simulink model "SolverSS_TestBed"  (R2012b)
settings: Solver=FixedStepDiscrete  StartTime=0.0  StopTime=100  FixedStep=1  RelTol=1e-3
libraries: Lib_Solve_SSNRSolverJC_TMATS x1
settings Model: Creator=jwchapm2  LastModifiedBy=jwchapm2

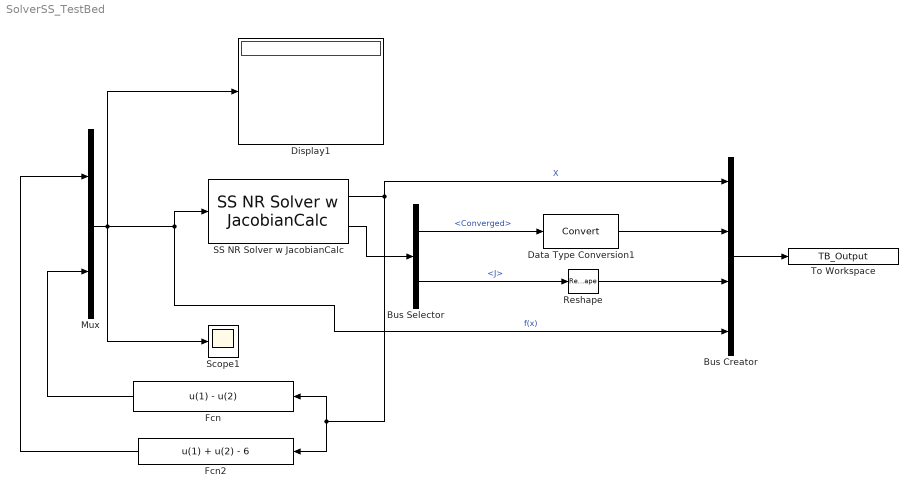
== system SolverSS_TestBed ==
  Bus Creator : BusCreator
  Bus Selector : BusSelector  OutputSignals=Converged,J
  Data Type Conversion1 : DataTypeConversion
  Display1 : Display
  Fcn : Fcn  Expr=u(1) - u(2)
  Fcn2 : Fcn  Expr=u(1) + u(2) - 6
  Mux : Mux  Inputs=2
  Reshape : Reshape
  SS NR Solver w JacobianCalc : Lib_Solve_SSNRSolverJC_TMATS/SS NR Solver w JacobianCalc  SJac_Per_M=MWS.SolverSS.Per  SNR_IC_M=MWS.SolverSS.IC  SNR_DX_M=MWS.SolverSS.dX  SJacobianAttempts_M=MWS.SolverSS.Jatm  Cond_Limits_M=MWS.SolverSS.Cond_Lim
  Scope1 : Scope
  To Workspace : ToWorkspace  VariableName=TB_Output  SampleTime=-1
  wires:
  Mux/1 -> Scope1/1, Display1/1, Bus Creator/4, SS NR Solver w JacobianCalc/1  "f(x)"
  SS NR Solver w JacobianCalc/1 -> Fcn2/1, Fcn/1, Bus Creator/1  "X"
  Bus Creator/1 -> To Workspace/1
  Fcn/1 -> Mux/2
  Fcn2/1 -> Mux/1
  SS NR Solver w JacobianCalc/2 -> Bus Selector/1
  Bus Selector/1 -> Data Type Conversion1/1  "<Converged>"
  Bus Selector/2 -> Reshape/1  "<J>"
  Data Type Conversion1/1 -> Bus Creator/2
  Reshape/1 -> Bus Creator/3
